simulink model "VehicleBody6DOFSSC"  (R2026b)
settings: Solver=VariableStepAuto
undefined symbols (not defined in the file): EnvAirDen, PlntVehAeroDragCff, PlntVehAeroFrntArea, PlntVehAeroLiftCff, PlntVehCGHgtAxl, PlntVehDstCGFrntAxl, PlntVehDstCGRearAxl, PlntVehInitLatPos, PlntVehInitVertPos, PlntVehMass, PlntVehMultiBody, PlntVehPitchMomentInertia, PlntVehRollMomentInertia, PlntVehTrckWdth, PlntVehYawMomentInertia, X, Y, Z
libraries: nesl_utility x68, sm_lib x60, sharedtransform x22, fl_lib x6, vehdynlibeomcommon x1, autolibutils x1
(part 2 of 3)

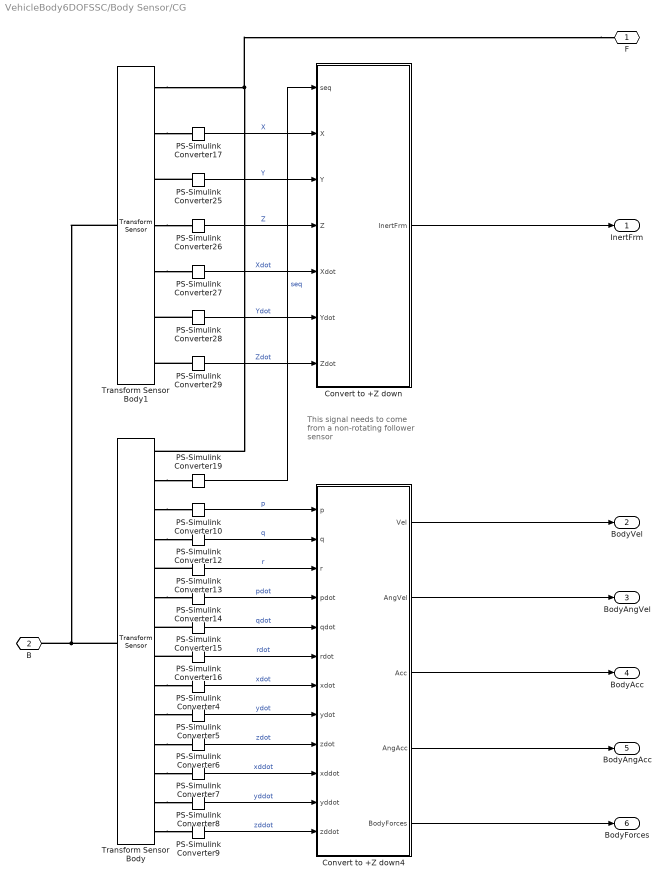
== system VehicleBody6DOFSSC/Body Sensor/CG ==
  note: This signal needs to come
      | from a non-rotating follower
      | sensor
  Convert to +Z down : Subsystem
  Convert to +Z down4 : Subsystem
  PS-Simulink Converter10 : nesl_utility/PS-Simulink Converter  PhysicalDomain=network_engine_domain  SubClassName=ps_output  LeftPortType=input  RightPortType=output  PseudoPeriodic=off  Frequencies=[]  VectorFormat=1-D array  Unit=rad/s  AffineConversion=off
  PS-Simulink Converter12 : nesl_utility/PS-Simulink Converter  PhysicalDomain=network_engine_domain  SubClassName=ps_output  LeftPortType=input  RightPortType=output  PseudoPeriodic=off  Frequencies=[]  VectorFormat=1-D array  Unit=rad/s  AffineConversion=off
  PS-Simulink Converter13 : nesl_utility/PS-Simulink Converter  PhysicalDomain=network_engine_domain  SubClassName=ps_output  LeftPortType=input  RightPortType=output  PseudoPeriodic=off  Frequencies=[]  VectorFormat=1-D array  Unit=rad/s  AffineConversion=off
  PS-Simulink Converter14 : nesl_utility/PS-Simulink Converter  PhysicalDomain=network_engine_domain  SubClassName=ps_output  LeftPortType=input  RightPortType=output  PseudoPeriodic=off  Frequencies=[]  VectorFormat=1-D array  Unit=rad/s^2  AffineConversion=off
  PS-Simulink Converter15 : nesl_utility/PS-Simulink Converter  PhysicalDomain=network_engine_domain  SubClassName=ps_output  LeftPortType=input  RightPortType=output  PseudoPeriodic=off  Frequencies=[]  VectorFormat=1-D array  Unit=rad/s^2  AffineConversion=off
  PS-Simulink Converter16 : nesl_utility/PS-Simulink Converter  PhysicalDomain=network_engine_domain  SubClassName=ps_output  LeftPortType=input  RightPortType=output  PseudoPeriodic=off  Frequencies=[]  VectorFormat=1-D array  Unit=rad/s^2  AffineConversion=off
  PS-Simulink Converter17 : nesl_utility/PS-Simulink Converter  PhysicalDomain=network_engine_domain  SubClassName=ps_output  LeftPortType=input  RightPortType=output  PseudoPeriodic=off  Frequencies=[]  VectorFormat=1-D array  Unit=m  AffineConversion=off
  PS-Simulink Converter19 : nesl_utility/PS-Simulink Converter  PhysicalDomain=network_engine_domain  SubClassName=ps_output  LeftPortType=input  RightPortType=output  PseudoPeriodic=off  Frequencies=[]  VectorFormat=1-D array  Unit=rad  AffineConversion=off
  PS-Simulink Converter25 : nesl_utility/PS-Simulink Converter  PhysicalDomain=network_engine_domain  SubClassName=ps_output  LeftPortType=input  RightPortType=output  PseudoPeriodic=off  Frequencies=[]  VectorFormat=1-D array  Unit=m  AffineConversion=off
  PS-Simulink Converter26 : nesl_utility/PS-Simulink Converter  PhysicalDomain=network_engine_domain  SubClassName=ps_output  LeftPortType=input  RightPortType=output  PseudoPeriodic=off  Frequencies=[]  VectorFormat=1-D array  Unit=m  AffineConversion=off
  PS-Simulink Converter{4..6,27..29} (6 alike) : nesl_utility/PS-Simulink Converter  PhysicalDomain=network_engine_domain  SubClassName=ps_output  LeftPortType=input  RightPortType=output  PseudoPeriodic=off  Frequencies=[]  VectorFormat=1-D array  Unit=m/s  AffineConversion=off
  PS-Simulink Converter7 : nesl_utility/PS-Simulink Converter  PhysicalDomain=network_engine_domain  SubClassName=ps_output  LeftPortType=input  RightPortType=output  PseudoPeriodic=off  Frequencies=[]  VectorFormat=1-D array  Unit=m/s^2  AffineConversion=off
  PS-Simulink Converter8 : nesl_utility/PS-Simulink Converter  PhysicalDomain=network_engine_domain  SubClassName=ps_output  LeftPortType=input  RightPortType=output  PseudoPeriodic=off  Frequencies=[]  VectorFormat=1-D array  Unit=m/s^2  AffineConversion=off
  PS-Simulink Converter9 : nesl_utility/PS-Simulink Converter  PhysicalDomain=network_engine_domain  SubClassName=ps_output  LeftPortType=input  RightPortType=output  PseudoPeriodic=off  Frequencies=[]  VectorFormat=1-D array  Unit=m/s^2  AffineConversion=off
  Transform Sensor Body : sm_lib/Frames and Transforms/Transform Sensor  ObservationFrame=World  ExpressedInFrame=Follower  RotationSequence=ZYX  SenseAngle=off  SenseAxis=off  SenseQ=off  SenseR=off  SenseRotationSequence=on  SenseOmegaX=on  SenseOmegaY=on  SenseOmegaZ=on  SenseOmega=off  SenseQDot=off  SenseRDot=off  SenseRotationSequenceDot=off  SenseAlphaX=on  SenseAlphaY=on  SenseAlphaZ=on  SenseAlpha=off  SenseQDDot=off  SenseRDDot=off  SenseX=off  SenseY=off  SenseZ=off  SenseXYZ=off  SenseRad=off  SenseAzim=off  SenseDist=off  SenseInc=off  SenseXDot=on  SenseYDot=on  SenseZDot=on  SenseXYZDot=off  SenseRadDot=off  SenseAzimDot=off  SenseDistDot=off  SenseIncDot=off  SenseXDDot=on  SenseYDDot=on  SenseZDDot=on  SenseXYZDDot=off  SenseRadDDot=off  SenseAzimDDot=off  SenseDistDDot=off  SenseIncDDot=off
  Transform Sensor Body1 : sm_lib/Frames and Transforms/Transform Sensor  ObservationFrame=Base  ExpressedInFrame=Base  RotationSequence=ZYX  SenseAngle=off  SenseAxis=off  SenseQ=off  SenseR=off  SenseRotationSequence=off  SenseOmegaX=off  SenseOmegaY=off  SenseOmegaZ=off  SenseOmega=off  SenseQDot=off  SenseRDot=off  SenseRotationSequenceDot=off  SenseAlphaX=off  SenseAlphaY=off  SenseAlphaZ=off  SenseAlpha=off  SenseQDDot=off  SenseRDDot=off  SenseX=on  SenseY=on  SenseZ=on  SenseXYZ=off  SenseRad=off  SenseAzim=off  SenseDist=off  SenseInc=off  SenseXDot=on  SenseYDot=on  SenseZDot=on  SenseXYZDot=off  SenseRadDot=off  SenseAzimDot=off  SenseDistDot=off  SenseIncDot=off  SenseXDDot=off  SenseYDDot=off  SenseZDDot=off  SenseXYZDDot=off  SenseRadDDot=off  SenseAzimDDot=off  SenseDistDDot=off  SenseIncDDot=off
  F : PMIOPort  Side=Right
  B : PMIOPort  Port=2  Side=Left
  InertFrm : Outport
  BodyVel : Outport  Port=2
  BodyAngVel : Outport  Port=3
  BodyAcc : Outport  Port=4
  BodyAngAcc : Outport  Port=5
  BodyForces : Outport  Port=6
  wires:
  Convert to +Z down4/3(Acc) -> BodyAcc/1
  Convert to +Z down4/1(Vel) -> BodyVel/1
  Convert to +Z down4/4(AngAcc) -> BodyAngAcc/1
  Convert to +Z down4/5(BodyForces) -> BodyForces/1
  PS-Simulink Converter17/1 -> Convert to +Z down/2(X)  "X"
  PS-Simulink Converter25/1 -> Convert to +Z down/3(Y)  "Y"
  PS-Simulink Converter7/1 -> Convert to +Z down4/10(xddot)  "xddot"
  PS-Simulink Converter14/1 -> Convert to +Z down4/4(pdot)  "pdot"
  Convert to +Z down4/2(AngVel) -> BodyAngVel/1
  PS-Simulink Converter5/1 -> Convert to +Z down4/8(ydot)  "ydot"
  PS-Simulink Converter28/1 -> Convert to +Z down/6(Ydot)  "Ydot"
  PS-Simulink Converter10/1 -> Convert to +Z down4/1(p)  "p"
  PS-Simulink Converter27/1 -> Convert to +Z down/5(Xdot)  "Xdot"
  PS-Simulink Converter12/1 -> Convert to +Z down4/2(q)  "q"
  PS-Simulink Converter4/1 -> Convert to +Z down4/7(xdot)  "xdot"
  PS-Simulink Converter29/1 -> Convert to +Z down/7(Zdot)  "Zdot"
  PS-Simulink Converter13/1 -> Convert to +Z down4/3(r)  "r"
  PS-Simulink Converter6/1 -> Convert to +Z down4/9(zdot)  "zdot"
  PS-Simulink Converter26/1 -> Convert to +Z down/4(Z)  "Z"
  Convert to +Z down/1(InertFrm) -> InertFrm/1
  PS-Simulink Converter9/1 -> Convert to +Z down4/12(zddot)  "zddot"
  PS-Simulink Converter16/1 -> Convert to +Z down4/6(rdot)  "rdot"
  PS-Simulink Converter19/1 -> Convert to +Z down/1(seq)  "seq"
  PS-Simulink Converter15/1 -> Convert to +Z down4/5(qdot)  "qdot"
  PS-Simulink Converter8/1 -> Convert to +Z down4/11(yddot)  "yddot"
  connections:
  PS-Simulink Converter29/LConn1 -- Transform Sensor Body1/RConn7
  Transform Sensor Body/RConn6 -- PS-Simulink Converter14/LConn1
  Transform Sensor Body/RConn10 -- PS-Simulink Converter5/LConn1
  Transform Sensor Body1/RConn5 -- PS-Simulink Converter27/LConn1
  Transform Sensor Body/RConn12 -- PS-Simulink Converter7/LConn1
  PS-Simulink Converter25/LConn1 -- Transform Sensor Body1/RConn3
  F/RConn1 -- Transform Sensor Body/RConn1 -- Transform Sensor Body1/RConn1
  Transform Sensor Body/RConn4 -- PS-Simulink Converter12/LConn1
  Transform Sensor Body/RConn14 -- PS-Simulink Converter9/LConn1
  PS-Simulink Converter16/LConn1 -- Transform Sensor Body/RConn8
  Transform Sensor Body/RConn13 -- PS-Simulink Converter8/LConn1
  Transform Sensor Body/RConn9 -- PS-Simulink Converter4/LConn1
  PS-Simulink Converter28/LConn1 -- Transform Sensor Body1/RConn6
  Transform Sensor Body1/RConn2 -- PS-Simulink Converter17/LConn1
  Transform Sensor Body/RConn11 -- PS-Simulink Converter6/LConn1
  Transform Sensor Body/RConn2 -- PS-Simulink Converter19/LConn1
  Transform Sensor Body1/RConn4 -- PS-Simulink Converter26/LConn1
  Transform Sensor Body1/LConn1 -- Transform Sensor Body/LConn1 -- B/RConn1
  Transform Sensor Body/RConn3 -- PS-Simulink Converter10/LConn1
  PS-Simulink Converter15/LConn1 -- Transform Sensor Body/RConn7
  PS-Simulink Converter13/LConn1 -- Transform Sensor Body/RConn5

== system VehicleBody6DOFSSC/Body Sensor/Drag Power Calculation ==
  Fdrag : Inport
  Vel : Inport  Port=2
  Abs1 : Abs  ZeroCross=off  SaturateOnIntegerOverflow=off
  Bus Selector : BusSelector  OutputSignals=Fdragx,Fdragz
  Bus Selector5 : BusSelector  OutputSignals=xdot,ydot,zdot  OutputAsBus=on
  Constant : Constant  Value=0  SampleTime=-1
  Product9 : Product
  Signal Specification : SignalSpecification  Unit=W
  Sum of Elements1 : Sum  Inputs=+
  Vector Concatenate : Concatenate  NumInputs=3
  DragPwr : Outport
  wires:
  Constant/1 -> Vector Concatenate/2
  Bus Selector/2 -> Vector Concatenate/3  "<Fdragz>"
  Bus Selector/1 -> Vector Concatenate/1  "<Fdragx>"
  Fdrag/1 -> Bus Selector/1
  Vel/1 -> Bus Selector5/1
  Sum of Elements1/1 -> Signal Specification/1
  Product9/1 -> Abs1/1
  Bus Selector5/1 -> Product9/2
  Vector Concatenate/1 -> Product9/1
  Abs1/1 -> Sum of Elements1/1
  Signal Specification/1 -> DragPwr/1

== system VehicleBody6DOFSSC/Body Sensor/FLAxle ==
  Convert to +Z down1 : Subsystem
  Convert to +Z down2 : Subsystem
  PS-Simulink Converter11 : nesl_utility/PS-Simulink Converter  PhysicalDomain=network_engine_domain  SubClassName=ps_output  LeftPortType=input  RightPortType=output  PseudoPeriodic=off  Frequencies=[]  VectorFormat=1-D array  Unit=m  AffineConversion=off
  PS-Simulink Converter18 : nesl_utility/PS-Simulink Converter  PhysicalDomain=network_engine_domain  SubClassName=ps_output  LeftPortType=input  RightPortType=output  PseudoPeriodic=off  Frequencies=[]  VectorFormat=1-D array  Unit=m  AffineConversion=off
  PS-Simulink Converter20 : nesl_utility/PS-Simulink Converter  PhysicalDomain=network_engine_domain  SubClassName=ps_output  LeftPortType=input  RightPortType=output  PseudoPeriodic=off  Frequencies=[]  VectorFormat=1-D array  Unit=m  AffineConversion=off
  PS-Simulink Converter{4..6,21..23} (6 alike) : nesl_utility/PS-Simulink Converter  PhysicalDomain=network_engine_domain  SubClassName=ps_output  LeftPortType=input  RightPortType=output  PseudoPeriodic=off  Frequencies=[]  VectorFormat=1-D array  Unit=m/s  AffineConversion=off
  Transform Sensor : sm_lib/Frames and Transforms/Transform Sensor  ObservationFrame=Base  ExpressedInFrame=Base  RotationSequence=ZYX  SenseAngle=off  SenseAxis=off  SenseQ=off  SenseR=off  SenseRotationSequence=off  SenseOmegaX=off  SenseOmegaY=off  SenseOmegaZ=off  SenseOmega=off  SenseQDot=off  SenseRDot=off  SenseRotationSequenceDot=off  SenseAlphaX=off  SenseAlphaY=off  SenseAlphaZ=off  SenseAlpha=off  SenseQDDot=off  SenseRDDot=off  SenseX=on  SenseY=on  SenseZ=on  SenseXYZ=off  SenseRad=off  SenseAzim=off  SenseDist=off  SenseInc=off  SenseXDot=on  SenseYDot=on  SenseZDot=on  SenseXYZDot=off  SenseRadDot=off  SenseAzimDot=off  SenseDistDot=off  SenseIncDot=off  SenseXDDot=off  SenseYDDot=off  SenseZDDot=off  SenseXYZDDot=off  SenseRadDDot=off  SenseAzimDDot=off  SenseDistDDot=off  SenseIncDDot=off
  Transform Sensor1 : sm_lib/Frames and Transforms/Transform Sensor  ObservationFrame=World  ExpressedInFrame=Follower  RotationSequence=ZYX  SenseAngle=off  SenseAxis=off  SenseQ=off  SenseR=off  SenseRotationSequence=off  SenseOmegaX=off  SenseOmegaY=off  SenseOmegaZ=off  SenseOmega=off  SenseQDot=off  SenseRDot=off  SenseRotationSequenceDot=off  SenseAlphaX=off  SenseAlphaY=off  SenseAlphaZ=off  SenseAlpha=off  SenseQDDot=off  SenseRDDot=off  SenseX=off  SenseY=off  SenseZ=off  SenseXYZ=off  SenseRad=off  SenseAzim=off  SenseDist=off  SenseInc=off  SenseXDot=on  SenseYDot=on  SenseZDot=on  SenseXYZDot=off  SenseRadDot=off  SenseAzimDot=off  SenseDistDot=off  SenseIncDot=off  SenseXDDot=off  SenseYDDot=off  SenseZDDot=off  SenseXYZDDot=off  SenseRadDDot=off  SenseAzimDDot=off  SenseDistDDot=off  SenseIncDDot=off
  F : PMIOPort  Side=Right
  B : PMIOPort  Port=2  Side=Left
  Inert : Outport
  Body : Outport  Port=2
  wires:
  Convert to +Z down2/1(Inert) -> Inert/1
  PS-Simulink Converter4/1 -> Convert to +Z down1/1(Xdot)  "xdot"
  PS-Simulink Converter5/1 -> Convert to +Z down1/2(Ydot)  "ydot"
  PS-Simulink Converter6/1 -> Convert to +Z down1/3(Zdot)  "zdot"
  Convert to +Z down1/1(Body) -> Body/1
  PS-Simulink Converter23/1 -> Convert to +Z down2/6(Zdot)  "Zdot"
  PS-Simulink Converter11/1 -> Convert to +Z down2/1(X)  "X"
  PS-Simulink Converter20/1 -> Convert to +Z down2/3(Z)  "Z"
  PS-Simulink Converter18/1 -> Convert to +Z down2/2(Y)  "Y"
  PS-Simulink Converter22/1 -> Convert to +Z down2/5(Ydot)  "Ydot"
  PS-Simulink Converter21/1 -> Convert to +Z down2/4(Xdot)  "Xdot"
  connections:
  Transform Sensor1/RConn4 -- PS-Simulink Converter6/LConn1
  Transform Sensor1/RConn3 -- PS-Simulink Converter5/LConn1
  Transform Sensor1/RConn2 -- PS-Simulink Converter4/LConn1
  Transform Sensor1/LConn1 -- Transform Sensor/LConn1 -- B/RConn1
  Transform Sensor1/RConn1 -- F/RConn1 -- Transform Sensor/RConn1
  Transform Sensor/RConn3 -- PS-Simulink Converter18/LConn1
  Transform Sensor/RConn4 -- PS-Simulink Converter20/LConn1
  Transform Sensor/RConn5 -- PS-Simulink Converter21/LConn1
  Transform Sensor/RConn2 -- PS-Simulink Converter11/LConn1
  Transform Sensor/RConn6 -- PS-Simulink Converter22/LConn1
  Transform Sensor/RConn7 -- PS-Simulink Converter23/LConn1

== system VehicleBody6DOFSSC/Body Sensor/FRAxle ==
  Convert to +Z down1 : Subsystem
  Convert to +Z down2 : Subsystem
  PS-Simulink Converter11 : nesl_utility/PS-Simulink Converter  PhysicalDomain=network_engine_domain  SubClassName=ps_output  LeftPortType=input  RightPortType=output  PseudoPeriodic=off  Frequencies=[]  VectorFormat=1-D array  Unit=m  AffineConversion=off
  PS-Simulink Converter18 : nesl_utility/PS-Simulink Converter  PhysicalDomain=network_engine_domain  SubClassName=ps_output  LeftPortType=input  RightPortType=output  PseudoPeriodic=off  Frequencies=[]  VectorFormat=1-D array  Unit=m  AffineConversion=off
  PS-Simulink Converter20 : nesl_utility/PS-Simulink Converter  PhysicalDomain=network_engine_domain  SubClassName=ps_output  LeftPortType=input  RightPortType=output  PseudoPeriodic=off  Frequencies=[]  VectorFormat=1-D array  Unit=m  AffineConversion=off
  PS-Simulink Converter{4..6,21..23} (6 alike) : nesl_utility/PS-Simulink Converter  PhysicalDomain=network_engine_domain  SubClassName=ps_output  LeftPortType=input  RightPortType=output  PseudoPeriodic=off  Frequencies=[]  VectorFormat=1-D array  Unit=m/s  AffineConversion=off
  Transform Sensor : sm_lib/Frames and Transforms/Transform Sensor  ObservationFrame=Base  ExpressedInFrame=Base  RotationSequence=ZYX  SenseAngle=off  SenseAxis=off  SenseQ=off  SenseR=off  SenseRotationSequence=off  SenseOmegaX=off  SenseOmegaY=off  SenseOmegaZ=off  SenseOmega=off  SenseQDot=off  SenseRDot=off  SenseRotationSequenceDot=off  SenseAlphaX=off  SenseAlphaY=off  SenseAlphaZ=off  SenseAlpha=off  SenseQDDot=off  SenseRDDot=off  SenseX=on  SenseY=on  SenseZ=on  SenseXYZ=off  SenseRad=off  SenseAzim=off  SenseDist=off  SenseInc=off  SenseXDot=on  SenseYDot=on  SenseZDot=on  SenseXYZDot=off  SenseRadDot=off  SenseAzimDot=off  SenseDistDot=off  SenseIncDot=off  SenseXDDot=off  SenseYDDot=off  SenseZDDot=off  SenseXYZDDot=off  SenseRadDDot=off  SenseAzimDDot=off  SenseDistDDot=off  SenseIncDDot=off
  Transform Sensor1 : sm_lib/Frames and Transforms/Transform Sensor  ObservationFrame=World  ExpressedInFrame=Follower  RotationSequence=ZYX  SenseAngle=off  SenseAxis=off  SenseQ=off  SenseR=off  SenseRotationSequence=off  SenseOmegaX=off  SenseOmegaY=off  SenseOmegaZ=off  SenseOmega=off  SenseQDot=off  SenseRDot=off  SenseRotationSequenceDot=off  SenseAlphaX=off  SenseAlphaY=off  SenseAlphaZ=off  SenseAlpha=off  SenseQDDot=off  SenseRDDot=off  SenseX=off  SenseY=off  SenseZ=off  SenseXYZ=off  SenseRad=off  SenseAzim=off  SenseDist=off  SenseInc=off  SenseXDot=on  SenseYDot=on  SenseZDot=on  SenseXYZDot=off  SenseRadDot=off  SenseAzimDot=off  SenseDistDot=off  SenseIncDot=off  SenseXDDot=off  SenseYDDot=off  SenseZDDot=off  SenseXYZDDot=off  SenseRadDDot=off  SenseAzimDDot=off  SenseDistDDot=off  SenseIncDDot=off
  F : PMIOPort  Side=Right
  B : PMIOPort  Port=2  Side=Left
  Inert : Outport
  Body : Outport  Port=2
  wires:
  PS-Simulink Converter21/1 -> Convert to +Z down2/4(Xdot)  "Xdot"
  PS-Simulink Converter22/1 -> Convert to +Z down2/5(Ydot)  "Ydot"
  PS-Simulink Converter18/1 -> Convert to +Z down2/2(Y)  "Y"
  PS-Simulink Converter20/1 -> Convert to +Z down2/3(Z)  "Z"
  PS-Simulink Converter11/1 -> Convert to +Z down2/1(X)  "X"
  PS-Simulink Converter23/1 -> Convert to +Z down2/6(Zdot)  "Zdot"
  Convert to +Z down1/1(Body) -> Body/1
  PS-Simulink Converter6/1 -> Convert to +Z down1/3(Zdot)  "zdot"
  PS-Simulink Converter5/1 -> Convert to +Z down1/2(Ydot)  "ydot"
  PS-Simulink Converter4/1 -> Convert to +Z down1/1(Xdot)  "xdot"
  Convert to +Z down2/1(Inert) -> Inert/1
  connections:
  Transform Sensor/RConn7 -- PS-Simulink Converter23/LConn1
  Transform Sensor/RConn6 -- PS-Simulink Converter22/LConn1
  Transform Sensor/RConn2 -- PS-Simulink Converter11/LConn1
  Transform Sensor/RConn5 -- PS-Simulink Converter21/LConn1
  Transform Sensor/RConn4 -- PS-Simulink Converter20/LConn1
  Transform Sensor/RConn3 -- PS-Simulink Converter18/LConn1
  Transform Sensor/RConn1 -- F/RConn1 -- Transform Sensor1/RConn1
  B/RConn1 -- Transform Sensor/LConn1 -- Transform Sensor1/LConn1
  Transform Sensor1/RConn2 -- PS-Simulink Converter4/LConn1
  Transform Sensor1/RConn3 -- PS-Simulink Converter5/LConn1
  Transform Sensor1/RConn4 -- PS-Simulink Converter6/LConn1

== system VehicleBody6DOFSSC/Body Sensor/Geom ==
  Convert to +Z down1 : Subsystem
  Convert to +Z down2 : Subsystem
  PS-Simulink Converter11 : nesl_utility/PS-Simulink Converter  PhysicalDomain=network_engine_domain  SubClassName=ps_output  LeftPortType=input  RightPortType=output  PseudoPeriodic=off  Frequencies=[]  VectorFormat=1-D array  Unit=m  AffineConversion=off
  PS-Simulink Converter18 : nesl_utility/PS-Simulink Converter  PhysicalDomain=network_engine_domain  SubClassName=ps_output  LeftPortType=input  RightPortType=output  PseudoPeriodic=off  Frequencies=[]  VectorFormat=1-D array  Unit=m  AffineConversion=off
  PS-Simulink Converter20 : nesl_utility/PS-Simulink Converter  PhysicalDomain=network_engine_domain  SubClassName=ps_output  LeftPortType=input  RightPortType=output  PseudoPeriodic=off  Frequencies=[]  VectorFormat=1-D array  Unit=m  AffineConversion=off
  PS-Simulink Converter{4..6,21..23} (6 alike) : nesl_utility/PS-Simulink Converter  PhysicalDomain=network_engine_domain  SubClassName=ps_output  LeftPortType=input  RightPortType=output  PseudoPeriodic=off  Frequencies=[]  VectorFormat=1-D array  Unit=m/s  AffineConversion=off
  Transform Sensor : sm_lib/Frames and Transforms/Transform Sensor  ObservationFrame=Base  ExpressedInFrame=Base  RotationSequence=ZYX  SenseAngle=off  SenseAxis=off  SenseQ=off  SenseR=off  SenseRotationSequence=off  SenseOmegaX=off  SenseOmegaY=off  SenseOmegaZ=off  SenseOmega=off  SenseQDot=off  SenseRDot=off  SenseRotationSequenceDot=off  SenseAlphaX=off  SenseAlphaY=off  SenseAlphaZ=off  SenseAlpha=off  SenseQDDot=off  SenseRDDot=off  SenseX=on  SenseY=on  SenseZ=on  SenseXYZ=off  SenseRad=off  SenseAzim=off  SenseDist=off  SenseInc=off  SenseXDot=on  SenseYDot=on  SenseZDot=on  SenseXYZDot=off  SenseRadDot=off  SenseAzimDot=off  SenseDistDot=off  SenseIncDot=off  SenseXDDot=off  SenseYDDot=off  SenseZDDot=off  SenseXYZDDot=off  SenseRadDDot=off  SenseAzimDDot=off  SenseDistDDot=off  SenseIncDDot=off
  Transform Sensor1 : sm_lib/Frames and Transforms/Transform Sensor  ObservationFrame=World  ExpressedInFrame=Follower  RotationSequence=ZYX  SenseAngle=off  SenseAxis=off  SenseQ=off  SenseR=off  SenseRotationSequence=off  SenseOmegaX=off  SenseOmegaY=off  SenseOmegaZ=off  SenseOmega=off  SenseQDot=off  SenseRDot=off  SenseRotationSequenceDot=off  SenseAlphaX=off  SenseAlphaY=off  SenseAlphaZ=off  SenseAlpha=off  SenseQDDot=off  SenseRDDot=off  SenseX=off  SenseY=off  SenseZ=off  SenseXYZ=off  SenseRad=off  SenseAzim=off  SenseDist=off  SenseInc=off  SenseXDot=on  SenseYDot=on  SenseZDot=on  SenseXYZDot=off  SenseRadDot=off  SenseAzimDot=off  SenseDistDot=off  SenseIncDot=off  SenseXDDot=off  SenseYDDot=off  SenseZDDot=off  SenseXYZDDot=off  SenseRadDDot=off  SenseAzimDDot=off  SenseDistDDot=off  SenseIncDDot=off
  F : PMIOPort  Side=Right
  B : PMIOPort  Port=2  Side=Left
  Inert : Outport
  Body : Outport  Port=2
  wires:
  Convert to +Z down2/1(Inert) -> Inert/1
  PS-Simulink Converter4/1 -> Convert to +Z down1/1(Xdot)  "xdot"
  PS-Simulink Converter5/1 -> Convert to +Z down1/2(Ydot)  "ydot"
  PS-Simulink Converter6/1 -> Convert to +Z down1/3(Zdot)  "zdot"
  Convert to +Z down1/1(Body) -> Body/1
  PS-Simulink Converter23/1 -> Convert to +Z down2/6(Zdot)  "Zdot"
  PS-Simulink Converter11/1 -> Convert to +Z down2/1(X)  "X"
  PS-Simulink Converter20/1 -> Convert to +Z down2/3(Z)  "Z"
  PS-Simulink Converter18/1 -> Convert to +Z down2/2(Y)  "Y"
  PS-Simulink Converter22/1 -> Convert to +Z down2/5(Ydot)  "Ydot"
  PS-Simulink Converter21/1 -> Convert to +Z down2/4(Xdot)  "Xdot"
  connections:
  Transform Sensor1/RConn4 -- PS-Simulink Converter6/LConn1
  Transform Sensor1/RConn3 -- PS-Simulink Converter5/LConn1
  Transform Sensor1/RConn2 -- PS-Simulink Converter4/LConn1
  Transform Sensor1/LConn1 -- Transform Sensor/LConn1 -- B/RConn1
  Transform Sensor1/RConn1 -- F/RConn1 -- Transform Sensor/RConn1
  Transform Sensor/RConn3 -- PS-Simulink Converter18/LConn1
  Transform Sensor/RConn4 -- PS-Simulink Converter20/LConn1
  Transform Sensor/RConn5 -- PS-Simulink Converter21/LConn1
  Transform Sensor/RConn2 -- PS-Simulink Converter11/LConn1
  Transform Sensor/RConn6 -- PS-Simulink Converter22/LConn1
  Transform Sensor/RConn7 -- PS-Simulink Converter23/LConn1

== system VehicleBody6DOFSSC/Body Sensor/RLAxle ==
  Convert to +Z down1 : Subsystem
  Convert to +Z down2 : Subsystem
  PS-Simulink Converter11 : nesl_utility/PS-Simulink Converter  PhysicalDomain=network_engine_domain  SubClassName=ps_output  LeftPortType=input  RightPortType=output  PseudoPeriodic=off  Frequencies=[]  VectorFormat=1-D array  Unit=m  AffineConversion=off
  PS-Simulink Converter18 : nesl_utility/PS-Simulink Converter  PhysicalDomain=network_engine_domain  SubClassName=ps_output  LeftPortType=input  RightPortType=output  PseudoPeriodic=off  Frequencies=[]  VectorFormat=1-D array  Unit=m  AffineConversion=off
  PS-Simulink Converter20 : nesl_utility/PS-Simulink Converter  PhysicalDomain=network_engine_domain  SubClassName=ps_output  LeftPortType=input  RightPortType=output  PseudoPeriodic=off  Frequencies=[]  VectorFormat=1-D array  Unit=m  AffineConversion=off
  PS-Simulink Converter{4..6,21..23} (6 alike) : nesl_utility/PS-Simulink Converter  PhysicalDomain=network_engine_domain  SubClassName=ps_output  LeftPortType=input  RightPortType=output  PseudoPeriodic=off  Frequencies=[]  VectorFormat=1-D array  Unit=m/s  AffineConversion=off
  Transform Sensor : sm_lib/Frames and Transforms/Transform Sensor  ObservationFrame=Base  ExpressedInFrame=Base  RotationSequence=ZYX  SenseAngle=off  SenseAxis=off  SenseQ=off  SenseR=off  SenseRotationSequence=off  SenseOmegaX=off  SenseOmegaY=off  SenseOmegaZ=off  SenseOmega=off  SenseQDot=off  SenseRDot=off  SenseRotationSequenceDot=off  SenseAlphaX=off  SenseAlphaY=off  SenseAlphaZ=off  SenseAlpha=off  SenseQDDot=off  SenseRDDot=off  SenseX=on  SenseY=on  SenseZ=on  SenseXYZ=off  SenseRad=off  SenseAzim=off  SenseDist=off  SenseInc=off  SenseXDot=on  SenseYDot=on  SenseZDot=on  SenseXYZDot=off  SenseRadDot=off  SenseAzimDot=off  SenseDistDot=off  SenseIncDot=off  SenseXDDot=off  SenseYDDot=off  SenseZDDot=off  SenseXYZDDot=off  SenseRadDDot=off  SenseAzimDDot=off  SenseDistDDot=off  SenseIncDDot=off
  Transform Sensor1 : sm_lib/Frames and Transforms/Transform Sensor  ObservationFrame=World  ExpressedInFrame=Follower  RotationSequence=ZYX  SenseAngle=off  SenseAxis=off  SenseQ=off  SenseR=off  SenseRotationSequence=off  SenseOmegaX=off  SenseOmegaY=off  SenseOmegaZ=off  SenseOmega=off  SenseQDot=off  SenseRDot=off  SenseRotationSequenceDot=off  SenseAlphaX=off  SenseAlphaY=off  SenseAlphaZ=off  SenseAlpha=off  SenseQDDot=off  SenseRDDot=off  SenseX=off  SenseY=off  SenseZ=off  SenseXYZ=off  SenseRad=off  SenseAzim=off  SenseDist=off  SenseInc=off  SenseXDot=on  SenseYDot=on  SenseZDot=on  SenseXYZDot=off  SenseRadDot=off  SenseAzimDot=off  SenseDistDot=off  SenseIncDot=off  SenseXDDot=off  SenseYDDot=off  SenseZDDot=off  SenseXYZDDot=off  SenseRadDDot=off  SenseAzimDDot=off  SenseDistDDot=off  SenseIncDDot=off
  F : PMIOPort  Side=Right
  B : PMIOPort  Port=2  Side=Left
  Inert : Outport
  Body : Outport  Port=2
  wires:
  Convert to +Z down2/1(Inert) -> Inert/1
  PS-Simulink Converter4/1 -> Convert to +Z down1/1(Xdot)  "xdot"
  PS-Simulink Converter5/1 -> Convert to +Z down1/2(Ydot)  "ydot"
  PS-Simulink Converter6/1 -> Convert to +Z down1/3(Zdot)  "zdot"
  Convert to +Z down1/1(Body) -> Body/1
  PS-Simulink Converter23/1 -> Convert to +Z down2/6(Zdot)  "Zdot"
  PS-Simulink Converter11/1 -> Convert to +Z down2/1(X)  "X"
  PS-Simulink Converter20/1 -> Convert to +Z down2/3(Z)  "Z"
  PS-Simulink Converter18/1 -> Convert to +Z down2/2(Y)  "Y"
  PS-Simulink Converter22/1 -> Convert to +Z down2/5(Ydot)  "Ydot"
  PS-Simulink Converter21/1 -> Convert to +Z down2/4(Xdot)  "Xdot"
  connections:
  Transform Sensor1/RConn4 -- PS-Simulink Converter6/LConn1
  Transform Sensor1/RConn3 -- PS-Simulink Converter5/LConn1
  Transform Sensor1/RConn2 -- PS-Simulink Converter4/LConn1
  Transform Sensor1/LConn1 -- Transform Sensor/LConn1 -- B/RConn1
  Transform Sensor1/RConn1 -- F/RConn1 -- Transform Sensor/RConn1
  Transform Sensor/RConn3 -- PS-Simulink Converter18/LConn1
  Transform Sensor/RConn4 -- PS-Simulink Converter20/LConn1
  Transform Sensor/RConn5 -- PS-Simulink Converter21/LConn1
  Transform Sensor/RConn2 -- PS-Simulink Converter11/LConn1
  Transform Sensor/RConn6 -- PS-Simulink Converter22/LConn1
  Transform Sensor/RConn7 -- PS-Simulink Converter23/LConn1

== system VehicleBody6DOFSSC/Body Sensor/RRAxle ==
  Convert to +Z down1 : Subsystem
  Convert to +Z down2 : Subsystem
  PS-Simulink Converter11 : nesl_utility/PS-Simulink Converter  PhysicalDomain=network_engine_domain  SubClassName=ps_output  LeftPortType=input  RightPortType=output  PseudoPeriodic=off  Frequencies=[]  VectorFormat=1-D array  Unit=m  AffineConversion=off
  PS-Simulink Converter18 : nesl_utility/PS-Simulink Converter  PhysicalDomain=network_engine_domain  SubClassName=ps_output  LeftPortType=input  RightPortType=output  PseudoPeriodic=off  Frequencies=[]  VectorFormat=1-D array  Unit=m  AffineConversion=off
  PS-Simulink Converter20 : nesl_utility/PS-Simulink Converter  PhysicalDomain=network_engine_domain  SubClassName=ps_output  LeftPortType=input  RightPortType=output  PseudoPeriodic=off  Frequencies=[]  VectorFormat=1-D array  Unit=m  AffineConversion=off
  PS-Simulink Converter{4..6,21..23} (6 alike) : nesl_utility/PS-Simulink Converter  PhysicalDomain=network_engine_domain  SubClassName=ps_output  LeftPortType=input  RightPortType=output  PseudoPeriodic=off  Frequencies=[]  VectorFormat=1-D array  Unit=m/s  AffineConversion=off
  Transform Sensor : sm_lib/Frames and Transforms/Transform Sensor  ObservationFrame=Base  ExpressedInFrame=Base  RotationSequence=ZYX  SenseAngle=off  SenseAxis=off  SenseQ=off  SenseR=off  SenseRotationSequence=off  SenseOmegaX=off  SenseOmegaY=off  SenseOmegaZ=off  SenseOmega=off  SenseQDot=off  SenseRDot=off  SenseRotationSequenceDot=off  SenseAlphaX=off  SenseAlphaY=off  SenseAlphaZ=off  SenseAlpha=off  SenseQDDot=off  SenseRDDot=off  SenseX=on  SenseY=on  SenseZ=on  SenseXYZ=off  SenseRad=off  SenseAzim=off  SenseDist=off  SenseInc=off  SenseXDot=on  SenseYDot=on  SenseZDot=on  SenseXYZDot=off  SenseRadDot=off  SenseAzimDot=off  SenseDistDot=off  SenseIncDot=off  SenseXDDot=off  SenseYDDot=off  SenseZDDot=off  SenseXYZDDot=off  SenseRadDDot=off  SenseAzimDDot=off  SenseDistDDot=off  SenseIncDDot=off
  Transform Sensor1 : sm_lib/Frames and Transforms/Transform Sensor  ObservationFrame=World  ExpressedInFrame=Follower  RotationSequence=ZYX  SenseAngle=off  SenseAxis=off  SenseQ=off  SenseR=off  SenseRotationSequence=off  SenseOmegaX=off  SenseOmegaY=off  SenseOmegaZ=off  SenseOmega=off  SenseQDot=off  SenseRDot=off  SenseRotationSequenceDot=off  SenseAlphaX=off  SenseAlphaY=off  SenseAlphaZ=off  SenseAlpha=off  SenseQDDot=off  SenseRDDot=off  SenseX=off  SenseY=off  SenseZ=off  SenseXYZ=off  SenseRad=off  SenseAzim=off  SenseDist=off  SenseInc=off  SenseXDot=on  SenseYDot=on  SenseZDot=on  SenseXYZDot=off  SenseRadDot=off  SenseAzimDot=off  SenseDistDot=off  SenseIncDot=off  SenseXDDot=off  SenseYDDot=off  SenseZDDot=off  SenseXYZDDot=off  SenseRadDDot=off  SenseAzimDDot=off  SenseDistDDot=off  SenseIncDDot=off
  F : PMIOPort  Side=Right
  B : PMIOPort  Port=2  Side=Left
  Inert : Outport
  Body : Outport  Port=2
  wires:
  PS-Simulink Converter21/1 -> Convert to +Z down2/4(Xdot)  "Xdot"
  PS-Simulink Converter22/1 -> Convert to +Z down2/5(Ydot)  "Ydot"
  PS-Simulink Converter18/1 -> Convert to +Z down2/2(Y)  "Y"
  PS-Simulink Converter20/1 -> Convert to +Z down2/3(Z)  "Z"
  PS-Simulink Converter11/1 -> Convert to +Z down2/1(X)  "X"
  PS-Simulink Converter23/1 -> Convert to +Z down2/6(Zdot)  "Zdot"
  Convert to +Z down1/1(Body) -> Body/1
  PS-Simulink Converter6/1 -> Convert to +Z down1/3(Zdot)  "zdot"
  PS-Simulink Converter5/1 -> Convert to +Z down1/2(Ydot)  "ydot"
  PS-Simulink Converter4/1 -> Convert to +Z down1/1(Xdot)  "xdot"
  Convert to +Z down2/1(Inert) -> Inert/1
  connections:
  Transform Sensor/RConn7 -- PS-Simulink Converter23/LConn1
  Transform Sensor/RConn6 -- PS-Simulink Converter22/LConn1
  Transform Sensor/RConn2 -- PS-Simulink Converter11/LConn1
  Transform Sensor/RConn5 -- PS-Simulink Converter21/LConn1
  Transform Sensor/RConn4 -- PS-Simulink Converter20/LConn1
  Transform Sensor/RConn3 -- PS-Simulink Converter18/LConn1
  Transform Sensor/RConn1 -- F/RConn1 -- Transform Sensor1/RConn1
  B/RConn1 -- Transform Sensor/LConn1 -- Transform Sensor1/LConn1
  Transform Sensor1/RConn2 -- PS-Simulink Converter4/LConn1
  Transform Sensor1/RConn3 -- PS-Simulink Converter5/LConn1
  Transform Sensor1/RConn4 -- PS-Simulink Converter6/LConn1

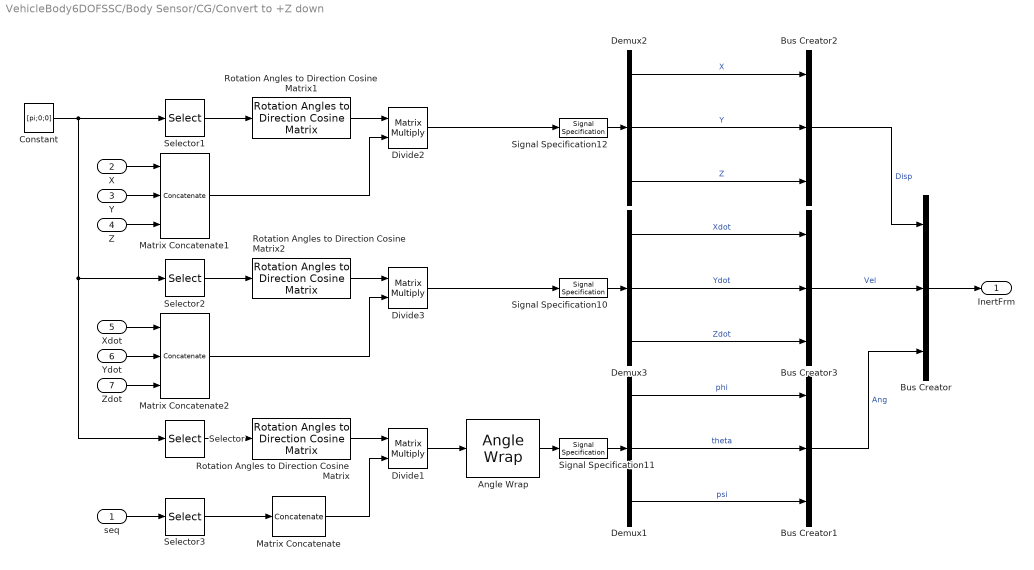
== system VehicleBody6DOFSSC/Body Sensor/CG/Convert to +Z down ==
  seq : Inport
  X : Inport  Port=2
  Y : Inport  Port=3
  Z : Inport  Port=4
  Xdot : Inport  Port=5
  Ydot : Inport  Port=6
  Zdot : Inport  Port=7
  Angle Wrap : vehdynlibeomcommon/6 DOF Generic Vehicle Body/SignalCollection/Angle Wrap  SystemSampleTime=-1  VariantControl=Variant1  LabelModeActiveChoice=Unwrap  VariantActivationTime=update diagram  EmptyChoice=off  PassThrough=off  PassThroughVariantControl=(default)  EmptyChoiceVariantControl=(default)  AllowFlexibleInterface=on  Latency=0  AutoFrameSizeCalculation=off
      link override Unwrap/Unwrap: aMode=2
  Bus Creator{,1..3} (4 alike) : BusCreator  Inputs=3
  Constant : Constant  Value=[pi;0;0]  SampleTime=-1
  Demux1 : Demux  Outputs=3
  Demux2 : Demux  Outputs=3
  Demux3 : Demux  Outputs=3
  Divide1 : Product  Inputs=**  Multiplication=Matrix(*)
  Divide2 : Product  Inputs=**  Multiplication=Matrix(*)
  Divide3 : Product  Inputs=**  Multiplication=Matrix(*)
  Matrix Concatenate : Concatenate  NumInputs=1  Mode=Multidimensional array
  Matrix Concatenate1 : Concatenate  NumInputs=3  Mode=Multidimensional array
  Matrix Concatenate2 : Concatenate  NumInputs=3  Mode=Multidimensional array
  Rotation Angles to Direction Cosine Matrix : sharedtransform/Rotation Angles to Direction Cosine Matrix  rotationOrder=ZYX  aMode=2
  Rotation Angles to Direction Cosine Matrix1 : sharedtransform/Rotation Angles to Direction Cosine Matrix  rotationOrder=ZYX  aMode=2
  Rotation Angles to Direction Cosine Matrix2 : sharedtransform/Rotation Angles to Direction Cosine Matrix  rotationOrder=ZYX  aMode=2
  Selector{,1..3} (4 alike) : Selector  InputPortWidth=3  IndexOptions=Index vector (dialog)  Indices=[3 2 1]  OutputSizes=1
  Signal Specification10 : SignalSpecification  Unit=m/s
  Signal Specification11 : SignalSpecification  Unit=rad
  Signal Specification12 : SignalSpecification  Unit=m
  InertFrm : Outport
  wires:
  Bus Creator1/1 -> Bus Creator/3  "Ang"
  Bus Creator2/1 -> Bus Creator/1  "Disp"
  Bus Creator3/1 -> Bus Creator/2  "Vel"
  Selector3/1 -> Matrix Concatenate/1
  seq/1 -> Selector3/1
  Signal Specification11/1 -> Demux1/1
  Demux1/1 -> Bus Creator1/1  "phi"
  Demux1/2 -> Bus Creator1/2  "theta"
  Angle Wrap/1 -> Signal Specification11/1
  Matrix Concatenate/1 -> Divide1/2
  Divide1/1 -> Angle Wrap/1
  Selector/1 -> Rotation Angles to Direction Cosine Matrix/1
  Rotation Angles to Direction Cosine Matrix/1 -> Divide1/1
  Demux2/2 -> Bus Creator2/2  "Y"
  Demux3/3 -> Bus Creator3/3  "Zdot"
  Demux2/3 -> Bus Creator2/3  "Z"
  Demux3/2 -> Bus Creator3/2  "Ydot"
  Demux3/1 -> Bus Creator3/1  "Xdot"
  Demux2/1 -> Bus Creator2/1  "X"
  Demux1/3 -> Bus Creator1/3  "psi"
  Matrix Concatenate1/1 -> Divide2/2
  X/1 -> Matrix Concatenate1/1
  Rotation Angles to Direction Cosine Matrix1/1 -> Divide2/1
  Selector1/1 -> Rotation Angles to Direction Cosine Matrix1/1
  Divide2/1 -> Signal Specification12/1
  Y/1 -> Matrix Concatenate1/2
  Z/1 -> Matrix Concatenate1/3
  Zdot/1 -> Matrix Concatenate2/3
  Ydot/1 -> Matrix Concatenate2/2
  Selector2/1 -> Rotation Angles to Direction Cosine Matrix2/1
  Rotation Angles to Direction Cosine Matrix2/1 -> Divide3/1
  Constant/1 -> Selector1/1, Selector2/1, Selector/1
  Xdot/1 -> Matrix Concatenate2/1
  Matrix Concatenate2/1 -> Divide3/2
  Divide3/1 -> Signal Specification10/1
  Bus Creator/1 -> InertFrm/1
  Signal Specification10/1 -> Demux3/1
  Signal Specification12/1 -> Demux2/1

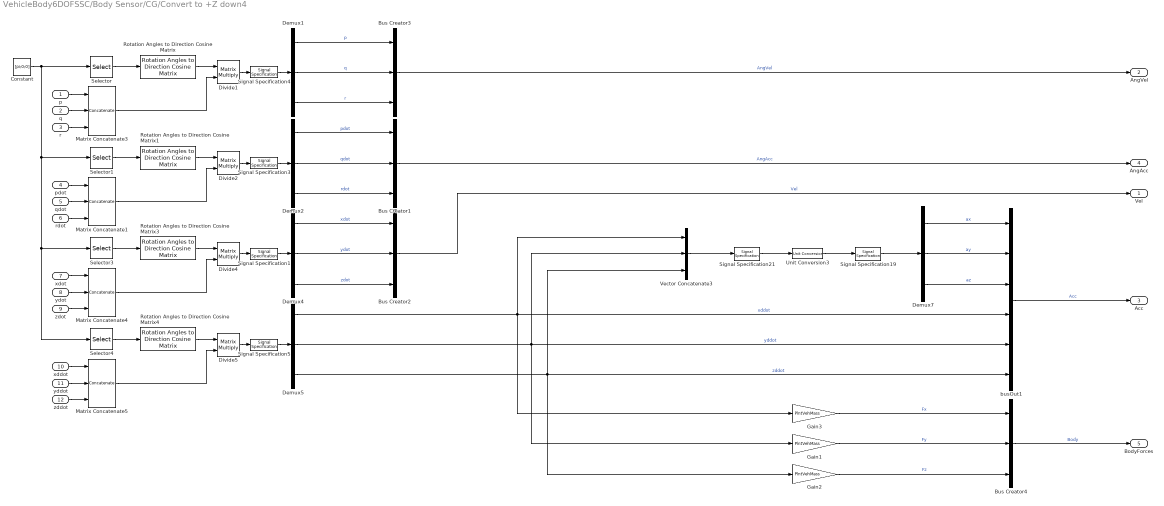
== system VehicleBody6DOFSSC/Body Sensor/CG/Convert to +Z down4 ==
  p : Inport
  q : Inport  Port=2
  r : Inport  Port=3
  pdot : Inport  Port=4
  qdot : Inport  Port=5
  rdot : Inport  Port=6
  xdot : Inport  Port=7
  ydot : Inport  Port=8
  zdot : Inport  Port=9
  xddot : Inport  Port=10
  yddot : Inport  Port=11
  zddot : Inport  Port=12
  Bus Creator{1..4} (4 alike) : BusCreator  Inputs=3
  Constant : Constant  Value=[pi;0;0]  SampleTime=-1
  Demux{1..2,4..5,7} (5 alike) : Demux  Outputs=3
  Divide{1..2,4..5} (4 alike) : Product  Inputs=**  Multiplication=Matrix(*)
  Gain1 : Gain  Gain=PlntVehMass
  Gain2 : Gain  Gain=PlntVehMass
  Gain3 : Gain  Gain=PlntVehMass
  Matrix Concatenate{1,3..5} (4 alike) : Concatenate  NumInputs=3  Mode=Multidimensional array
  Rotation Angles to Direction Cosine Matrix{,1,3..4} (4 alike) : sharedtransform/Rotation Angles to Direction Cosine Matrix  rotationOrder=ZYX  aMode=2
  Selector{,1,3..4} (4 alike) : Selector  InputPortWidth=3  IndexOptions=Index vector (dialog)  Indices=[3 2 1]  OutputSizes=1
  Signal Specification1 : SignalSpecification  Unit=m/s
  Signal Specification19 : SignalSpecification  Unit=gn
  Signal Specification21 : SignalSpecification  Unit=m/s^2
  Signal Specification3 : SignalSpecification  Unit=rad/s^2
  Signal Specification4 : SignalSpecification  Unit=rad/s
  Signal Specification5 : SignalSpecification  Unit=m/s^2
  Unit Conversion3 : UnitConversion
  Vector Concatenate3 : Concatenate  NumInputs=3
  busOut1 : BusCreator  Inputs=6
  Vel : Outport
  AngVel : Outport  Port=2
  Acc : Outport  Port=3
  AngAcc : Outport  Port=4
  BodyForces : Outport  Port=5
  wires:
  Bus Creator4/1 -> BodyForces/1  "Body"
  Gain3/1 -> Bus Creator4/1  "Fx"
  Gain1/1 -> Bus Creator4/2  "Fy"
  Gain2/1 -> Bus Creator4/3  "Fz"
  Bus Creator3/1 -> AngVel/1  "AngVel"
  Bus Creator1/1 -> AngAcc/1  "AngAcc"
  Bus Creator2/1 -> Vel/1  "Vel"
  busOut1/1 -> Acc/1  "Acc"
  Demux5/3 -> Gain2/1, busOut1/6, Vector Concatenate3/3  "zddot"
  Signal Specification19/1 -> Demux7/1
  Vector Concatenate3/1 -> Signal Specification21/1
  Demux7/3 -> busOut1/3  "az"
  Demux7/2 -> busOut1/2  "ay"
  Demux7/1 -> busOut1/1  "ax"
  Unit Conversion3/1 -> Signal Specification19/1
  Signal Specification21/1 -> Unit Conversion3/1
  Demux5/1 -> Vector Concatenate3/1, busOut1/4, Gain3/1  "xddot"
  Demux5/2 -> Vector Concatenate3/2, busOut1/5, Gain1/1  "yddot"
  Signal Specification4/1 -> Demux1/1
  Signal Specification3/1 -> Demux2/1
  Signal Specification1/1 -> Demux4/1
  Signal Specification5/1 -> Demux5/1
  Divide5/1 -> Signal Specification5/1
  zddot/1 -> Matrix Concatenate5/3
  yddot/1 -> Matrix Concatenate5/2
  Selector4/1 -> Rotation Angles to Direction Cosine Matrix4/1
  Rotation Angles to Direction Cosine Matrix4/1 -> Divide5/1
  Constant/1 -> Selector4/1, Selector3/1, Selector1/1, Selector/1
  xddot/1 -> Matrix Concatenate5/1
  Matrix Concatenate5/1 -> Divide5/2
  Divide4/1 -> Signal Specification1/1
  Matrix Concatenate4/1 -> Divide4/2
  xdot/1 -> Matrix Concatenate4/1
  Rotation Angles to Direction Cosine Matrix3/1 -> Divide4/1
  Selector3/1 -> Rotation Angles to Direction Cosine Matrix3/1
  ydot/1 -> Matrix Concatenate4/2
  zdot/1 -> Matrix Concatenate4/3
  q/1 -> Matrix Concatenate3/2
  r/1 -> Matrix Concatenate3/3
  p/1 -> Matrix Concatenate3/1
  Matrix Concatenate3/1 -> Divide1/2
  Demux4/3 -> Bus Creator2/3  "zdot"
  Demux4/2 -> Bus Creator2/2  "ydot"
  Demux4/1 -> Bus Creator2/1  "xdot"
  Demux2/3 -> Bus Creator1/3  "rdot"
  Demux2/2 -> Bus Creator1/2  "qdot"
  Demux2/1 -> Bus Creator1/1  "pdot"
  Demux1/3 -> Bus Creator3/3  "r"
  Demux1/2 -> Bus Creator3/2  "q"
  Demux1/1 -> Bus Creator3/1  "p"
  Selector/1 -> Rotation Angles to Direction Cosine Matrix/1
  Rotation Angles to Direction Cosine Matrix/1 -> Divide1/1
  Divide1/1 -> Signal Specification4/1
  Matrix Concatenate1/1 -> Divide2/2
  pdot/1 -> Matrix Concatenate1/1
  Rotation Angles to Direction Cosine Matrix1/1 -> Divide2/1
  Selector1/1 -> Rotation Angles to Direction Cosine Matrix1/1
  Divide2/1 -> Signal Specification3/1
  qdot/1 -> Matrix Concatenate1/2
  rdot/1 -> Matrix Concatenate1/3

== system VehicleBody6DOFSSC/Body Sensor/FLAxle/Convert to +Z down1 ==
  note: Setting constant
      | positions for Body Disp
      | because they do not
      | move relative to Body
      | Coordinate Frame
  Xdot : Inport
  Ydot : Inport  Port=2
  Zdot : Inport  Port=3
  Bus Creator : BusCreator  Inputs=2
  Bus Creator1 : BusCreator  Inputs=3
  Bus Creator2 : BusCreator  Inputs=3
  Constant : Constant  Value=[pi;0;0]  SampleTime=-1
  Constant1 : Constant  Value=PlntVehDstCGFrntAxl  SampleTime=-1
  Constant2 : Constant  Value=-PlntVehTrckWdth(1)/2  SampleTime=-1
  Constant3 : Constant  Value=PlntVehCGHgtAxl  SampleTime=-1
  Demux2 : Demux  Outputs=3
  Demux3 : Demux  Outputs=3
  Divide3 : Product  Inputs=**  Multiplication=Matrix(*)
  Matrix Concatenate2 : Concatenate  NumInputs=3  Mode=Multidimensional array
  Mux : Mux  Inputs=3
  Rotation Angles to Direction Cosine Matrix2 : sharedtransform/Rotation Angles to Direction Cosine Matrix  rotationOrder=ZYX  aMode=2
  Selector2 : Selector  InputPortWidth=3  IndexOptions=Index vector (dialog)  Indices=[3 2 1]  OutputSizes=1
  Signal Specification7 : SignalSpecification  Unit=m
  Signal Specification8 : SignalSpecification  Unit=m/s
  Body : Outport
  wires:
  Bus Creator1/1 -> Bus Creator/1  "Disp"
  Bus Creator/1 -> Body/1
  Bus Creator2/1 -> Bus Creator/2  "Vel"
  Constant3/1 -> Mux/3
  Constant1/1 -> Mux/1
  Constant2/1 -> Mux/2
  Mux/1 -> Signal Specification7/1
  Signal Specification8/1 -> Demux3/1
  Signal Specification7/1 -> Demux2/1
  Demux2/2 -> Bus Creator1/2  "y"
  Demux3/3 -> Bus Creator2/3  "zdot"
  Demux2/3 -> Bus Creator1/3  "z"
  Demux3/2 -> Bus Creator2/2  "ydot"
  Demux3/1 -> Bus Creator2/1  "xdot"
  Demux2/1 -> Bus Creator1/1  "x"
  Zdot/1 -> Matrix Concatenate2/3
  Ydot/1 -> Matrix Concatenate2/2
  Selector2/1 -> Rotation Angles to Direction Cosine Matrix2/1
  Rotation Angles to Direction Cosine Matrix2/1 -> Divide3/1
  Constant/1 -> Selector2/1
  Xdot/1 -> Matrix Concatenate2/1
  Matrix Concatenate2/1 -> Divide3/2
  Divide3/1 -> Signal Specification8/1

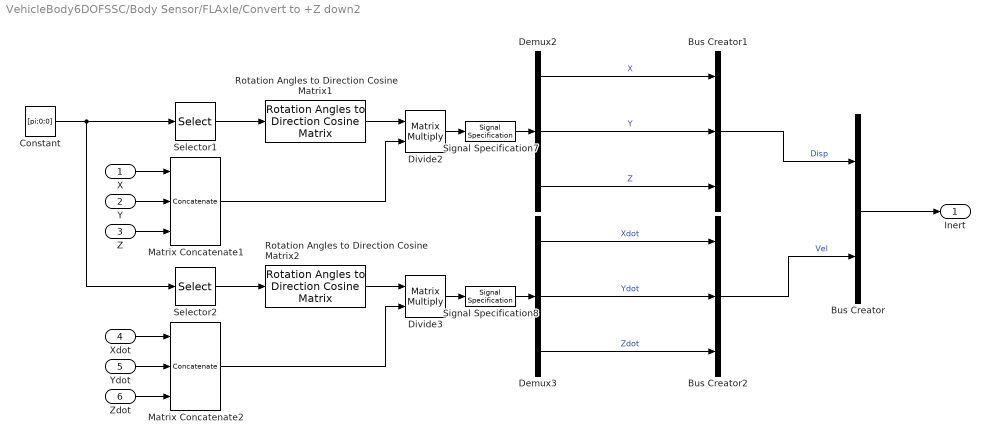
== system VehicleBody6DOFSSC/Body Sensor/FLAxle/Convert to +Z down2 ==
  X : Inport
  Y : Inport  Port=2
  Z : Inport  Port=3
  Xdot : Inport  Port=4
  Ydot : Inport  Port=5
  Zdot : Inport  Port=6
  Bus Creator : BusCreator  Inputs=2
  Bus Creator1 : BusCreator  Inputs=3
  Bus Creator2 : BusCreator  Inputs=3
  Constant : Constant  Value=[pi;0;0]  SampleTime=-1
  Demux2 : Demux  Outputs=3
  Demux3 : Demux  Outputs=3
  Divide2 : Product  Inputs=**  Multiplication=Matrix(*)
  Divide3 : Product  Inputs=**  Multiplication=Matrix(*)
  Matrix Concatenate1 : Concatenate  NumInputs=3  Mode=Multidimensional array
  Matrix Concatenate2 : Concatenate  NumInputs=3  Mode=Multidimensional array
  Rotation Angles to Direction Cosine Matrix1 : sharedtransform/Rotation Angles to Direction Cosine Matrix  rotationOrder=ZYX  aMode=2
  Rotation Angles to Direction Cosine Matrix2 : sharedtransform/Rotation Angles to Direction Cosine Matrix  rotationOrder=ZYX  aMode=2
  Selector1 : Selector  InputPortWidth=3  IndexOptions=Index vector (dialog)  Indices=[3 2 1]  OutputSizes=1
  Selector2 : Selector  InputPortWidth=3  IndexOptions=Index vector (dialog)  Indices=[3 2 1]  OutputSizes=1
  Signal Specification7 : SignalSpecification  Unit=m
  Signal Specification8 : SignalSpecification  Unit=m/s
  Inert : Outport
  wires:
  Bus Creator/1 -> Inert/1
  Bus Creator2/1 -> Bus Creator/2  "Vel"
  Bus Creator1/1 -> Bus Creator/1  "Disp"
  Divide3/1 -> Signal Specification8/1
  Matrix Concatenate2/1 -> Divide3/2
  Xdot/1 -> Matrix Concatenate2/1
  Constant/1 -> Selector1/1, Selector2/1
  Rotation Angles to Direction Cosine Matrix2/1 -> Divide3/1
  Selector2/1 -> Rotation Angles to Direction Cosine Matrix2/1
  Ydot/1 -> Matrix Concatenate2/2
  Zdot/1 -> Matrix Concatenate2/3
  Z/1 -> Matrix Concatenate1/3
  Y/1 -> Matrix Concatenate1/2
  Divide2/1 -> Signal Specification7/1
  Selector1/1 -> Rotation Angles to Direction Cosine Matrix1/1
  Rotation Angles to Direction Cosine Matrix1/1 -> Divide2/1
  X/1 -> Matrix Concatenate1/1
  Matrix Concatenate1/1 -> Divide2/2
  Demux2/1 -> Bus Creator1/1  "X"
  Demux3/1 -> Bus Creator2/1  "Xdot"
  Demux3/2 -> Bus Creator2/2  "Ydot"
  Demux2/3 -> Bus Creator1/3  "Z"
  Demux3/3 -> Bus Creator2/3  "Zdot"
  Demux2/2 -> Bus Creator1/2  "Y"
  Signal Specification7/1 -> Demux2/1
  Signal Specification8/1 -> Demux3/1

== system VehicleBody6DOFSSC/Body Sensor/FRAxle/Convert to +Z down1 ==
  note: Setting constant
      | positions for Body Disp
      | because they do not
      | move relative to Body
      | Coordinate Frame
  Xdot : Inport
  Ydot : Inport  Port=2
  Zdot : Inport  Port=3
  Bus Creator : BusCreator  Inputs=2
  Bus Creator1 : BusCreator  Inputs=3
  Bus Creator2 : BusCreator  Inputs=3
  Constant : Constant  Value=[pi;0;0]  SampleTime=-1
  Constant1 : Constant  Value=PlntVehDstCGFrntAxl  SampleTime=-1
  Constant2 : Constant  Value=PlntVehTrckWdth(1)/2  SampleTime=-1
  Constant3 : Constant  Value=PlntVehCGHgtAxl  SampleTime=-1
  Demux2 : Demux  Outputs=3
  Demux3 : Demux  Outputs=3
  Divide3 : Product  Inputs=**  Multiplication=Matrix(*)
  Matrix Concatenate2 : Concatenate  NumInputs=3  Mode=Multidimensional array
  Mux : Mux  Inputs=3
  Rotation Angles to Direction Cosine Matrix2 : sharedtransform/Rotation Angles to Direction Cosine Matrix  rotationOrder=ZYX  aMode=2
  Selector2 : Selector  InputPortWidth=3  IndexOptions=Index vector (dialog)  Indices=[3 2 1]  OutputSizes=1
  Signal Specification7 : SignalSpecification  Unit=m
  Signal Specification8 : SignalSpecification  Unit=m/s
  Body : Outport
  wires:
  Divide3/1 -> Signal Specification8/1
  Matrix Concatenate2/1 -> Divide3/2
  Xdot/1 -> Matrix Concatenate2/1
  Constant/1 -> Selector2/1
  Rotation Angles to Direction Cosine Matrix2/1 -> Divide3/1
  Selector2/1 -> Rotation Angles to Direction Cosine Matrix2/1
  Ydot/1 -> Matrix Concatenate2/2
  Zdot/1 -> Matrix Concatenate2/3
  Demux2/1 -> Bus Creator1/1  "x"
  Demux3/1 -> Bus Creator2/1  "xdot"
  Demux3/2 -> Bus Creator2/2  "ydot"
  Demux2/3 -> Bus Creator1/3  "z"
  Demux3/3 -> Bus Creator2/3  "zdot"
  Demux2/2 -> Bus Creator1/2  "y"
  Signal Specification7/1 -> Demux2/1
  Signal Specification8/1 -> Demux3/1
  Mux/1 -> Signal Specification7/1
  Constant2/1 -> Mux/2
  Constant1/1 -> Mux/1
  Constant3/1 -> Mux/3
  Bus Creator2/1 -> Bus Creator/2  "Vel"
  Bus Creator/1 -> Body/1
  Bus Creator1/1 -> Bus Creator/1  "Disp"

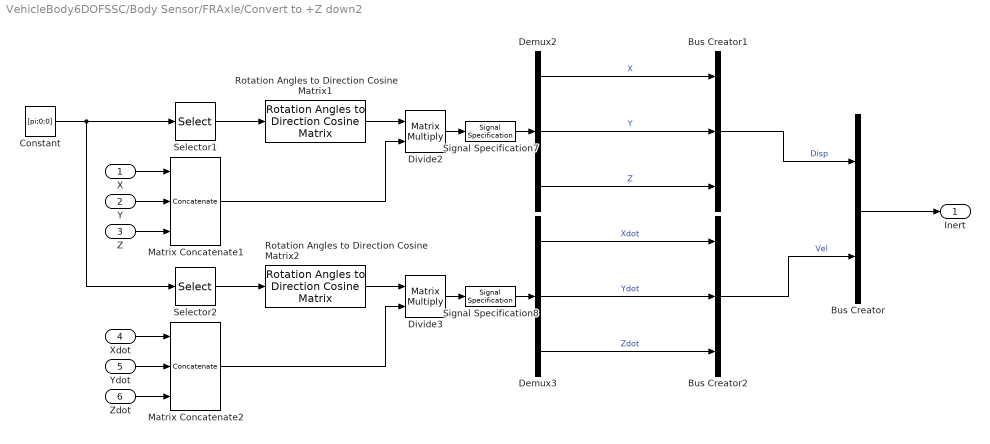
== system VehicleBody6DOFSSC/Body Sensor/FRAxle/Convert to +Z down2 ==
  X : Inport
  Y : Inport  Port=2
  Z : Inport  Port=3
  Xdot : Inport  Port=4
  Ydot : Inport  Port=5
  Zdot : Inport  Port=6
  Bus Creator : BusCreator  Inputs=2
  Bus Creator1 : BusCreator  Inputs=3
  Bus Creator2 : BusCreator  Inputs=3
  Constant : Constant  Value=[pi;0;0]  SampleTime=-1
  Demux2 : Demux  Outputs=3
  Demux3 : Demux  Outputs=3
  Divide2 : Product  Inputs=**  Multiplication=Matrix(*)
  Divide3 : Product  Inputs=**  Multiplication=Matrix(*)
  Matrix Concatenate1 : Concatenate  NumInputs=3  Mode=Multidimensional array
  Matrix Concatenate2 : Concatenate  NumInputs=3  Mode=Multidimensional array
  Rotation Angles to Direction Cosine Matrix1 : sharedtransform/Rotation Angles to Direction Cosine Matrix  rotationOrder=ZYX  aMode=2
  Rotation Angles to Direction Cosine Matrix2 : sharedtransform/Rotation Angles to Direction Cosine Matrix  rotationOrder=ZYX  aMode=2
  Selector1 : Selector  InputPortWidth=3  IndexOptions=Index vector (dialog)  Indices=[3 2 1]  OutputSizes=1
  Selector2 : Selector  InputPortWidth=3  IndexOptions=Index vector (dialog)  Indices=[3 2 1]  OutputSizes=1
  Signal Specification7 : SignalSpecification  Unit=m
  Signal Specification8 : SignalSpecification  Unit=m/s
  Inert : Outport
  wires:
  Signal Specification8/1 -> Demux3/1
  Signal Specification7/1 -> Demux2/1
  Demux2/2 -> Bus Creator1/2  "Y"
  Demux3/3 -> Bus Creator2/3  "Zdot"
  Demux2/3 -> Bus Creator1/3  "Z"
  Demux3/2 -> Bus Creator2/2  "Ydot"
  Demux3/1 -> Bus Creator2/1  "Xdot"
  Demux2/1 -> Bus Creator1/1  "X"
  Matrix Concatenate1/1 -> Divide2/2
  X/1 -> Matrix Concatenate1/1
  Rotation Angles to Direction Cosine Matrix1/1 -> Divide2/1
  Selector1/1 -> Rotation Angles to Direction Cosine Matrix1/1
  Divide2/1 -> Signal Specification7/1
  Y/1 -> Matrix Concatenate1/2
  Z/1 -> Matrix Concatenate1/3
  Zdot/1 -> Matrix Concatenate2/3
  Ydot/1 -> Matrix Concatenate2/2
  Selector2/1 -> Rotation Angles to Direction Cosine Matrix2/1
  Rotation Angles to Direction Cosine Matrix2/1 -> Divide3/1
  Constant/1 -> Selector2/1, Selector1/1
  Xdot/1 -> Matrix Concatenate2/1
  Matrix Concatenate2/1 -> Divide3/2
  Divide3/1 -> Signal Specification8/1
  Bus Creator1/1 -> Bus Creator/1  "Disp"
  Bus Creator2/1 -> Bus Creator/2  "Vel"
  Bus Creator/1 -> Inert/1
